simulink model "Aerial_Inspection_Octa_Rotor"  (R2021a)
settings: Solver=VariableStepAuto  StartTime=0.0  StopTime=2  RelTol=1e-3
model workspace: external: MATLAB File D:\MS_Control_Project\Simulation\SolidWorks output\Aerial_Inspection_Octa_Rotor_DataFile.m (data not in the file)
undefined symbols (not defined in the file or in its folder): Motor_data, params, servo_specs, smiData, stepper, Tm, X, Y, Z
libraries: sm_lib x810, nesl_utility x50, sharedtransform x1
(part 4 of 21)

== system Aerial_Inspection_Octa_Rotor/UAV/Device ==
  Device_1_RIGID : Subsystem
  Device_Box_1_RIGID : Subsystem
  F : PMIOPort  Side=Left
  connections:
  Device_1_RIGID/LConn1 -- Device_Box_1_RIGID/LConn1
  Device_Box_1_RIGID/LConn2 -- F/RConn1

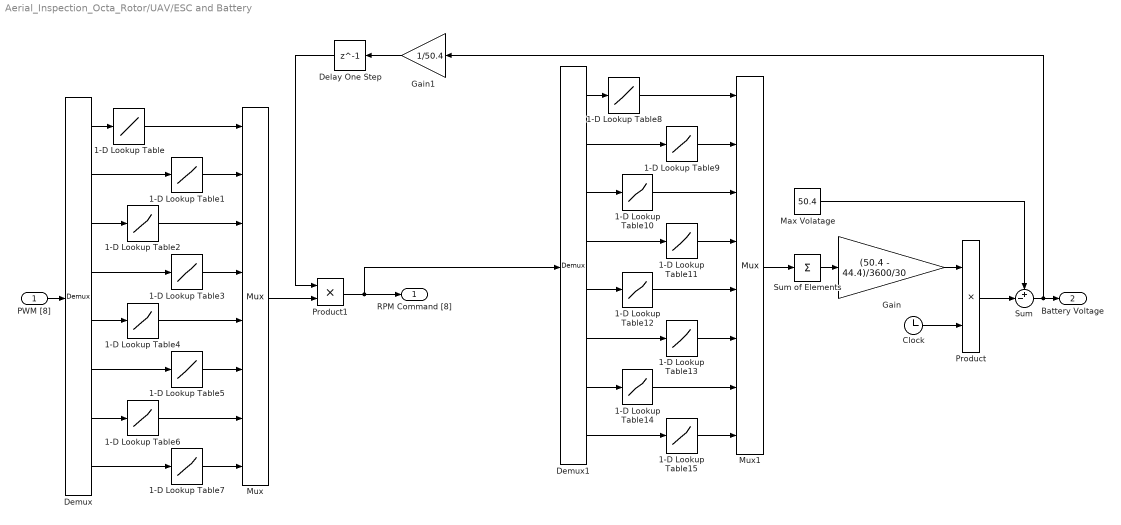
== system Aerial_Inspection_Octa_Rotor/UAV/ESC and Battery ==
  PWM [8] : Inport
  1-D Lookup Table{,1..7} (8 alike) : Lookup_n-D  NumberOfTableDimensions=1  BreakpointsForDimension1=[0;Motor_data.Throttle]  Table=[0;Motor_data.RPM]  InternalRulePriority=Speed  RndMeth=Simplest  InputSameDT=on
  1-D Lookup Table{8..15} (8 alike) : Lookup_n-D  NumberOfTableDimensions=1  BreakpointsForDimension1=[0;Motor_data.RPM]  Table=[0;Motor_data.Current]  InterpMethod=Cubic spline  ExtrapMethod=Cubic spline  InternalRulePriority=Speed  RndMeth=Simplest  InputSameDT=on
  Clock : Clock
  Delay One Step : Delay  DelayLength=1  InitialCondition=50.4
  Demux : Demux  Outputs=8
  Demux1 : Demux  Outputs=8
  Gain : Gain  Gain=(50.4 - 44.4)/3600/30
  Gain1 : Gain  Gain=1/50.4
  Max Volatage : Constant  Value=50.4
  Mux : Mux  Inputs=8
  Mux1 : Mux  Inputs=8
  Product : Product
  Product1 : Product
  Sum : Sum  Inputs=+-|
  Sum of Elements : Sum  Inputs=+
  RPM Command [8] : Outport
  Battery Voltage : Outport  Port=2
  wires:
  PWM [8]/1 -> Demux/1
  Demux/1 -> 1-D Lookup Table/1
  Demux/2 -> 1-D Lookup Table1/1
  Demux/3 -> 1-D Lookup Table2/1
  Demux/4 -> 1-D Lookup Table3/1
  Demux/5 -> 1-D Lookup Table4/1
  Demux/6 -> 1-D Lookup Table5/1
  Demux/7 -> 1-D Lookup Table6/1
  Demux/8 -> 1-D Lookup Table7/1
  1-D Lookup Table7/1 -> Mux/8
  1-D Lookup Table5/1 -> Mux/6
  1-D Lookup Table3/1 -> Mux/4
  1-D Lookup Table1/1 -> Mux/2
  1-D Lookup Table6/1 -> Mux/7
  1-D Lookup Table4/1 -> Mux/5
  1-D Lookup Table2/1 -> Mux/3
  1-D Lookup Table/1 -> Mux/1
  1-D Lookup Table8/1 -> Mux1/1
  1-D Lookup Table10/1 -> Mux1/3
  1-D Lookup Table12/1 -> Mux1/5
  1-D Lookup Table14/1 -> Mux1/7
  1-D Lookup Table9/1 -> Mux1/2
  1-D Lookup Table11/1 -> Mux1/4
  1-D Lookup Table13/1 -> Mux1/6
  1-D Lookup Table15/1 -> Mux1/8
  Demux1/8 -> 1-D Lookup Table15/1
  Demux1/7 -> 1-D Lookup Table14/1
  Demux1/6 -> 1-D Lookup Table13/1
  Demux1/5 -> 1-D Lookup Table12/1
  Demux1/4 -> 1-D Lookup Table11/1
  Demux1/3 -> 1-D Lookup Table10/1
  Demux1/2 -> 1-D Lookup Table9/1
  Demux1/1 -> 1-D Lookup Table8/1
  Mux1/1 -> Sum of Elements/1
  Sum of Elements/1 -> Gain/1
  Product/1 -> Sum/2
  Gain/1 -> Product/1
  Clock/1 -> Product/2
  Max Volatage/1 -> Sum/1
  Sum/1 -> Gain1/1, Battery Voltage/1
  Mux/1 -> Product1/2
  Product1/1 -> Demux1/1, RPM Command [8]/1
  Gain1/1 -> Delay One Step/1
  Delay One Step/1 -> Product1/1

== system Aerial_Inspection_Octa_Rotor/UAV/Landing Gear ==
  Front_lastic_1_RIGID : Subsystem
  Front_lastic_2_RIGID : Subsystem
  Landing_Gear_5_RIGID : Subsystem
  Rear_lastic_1_RIGID : Subsystem
  Rear_lastic_2_RIGID : Subsystem
  Revolute16 : sm_lib/Joints/Revolute Joint  JointMode=Normal  SenseConstraintForce=off  SenseConstraintForceX=off  SenseConstraintForceY=off  SenseConstraintForceZ=off  SenseConstraintTorque=off  SenseConstraintTorqueX=off  SenseConstraintTorqueY=off  SenseConstraintTorqueZ=off  SenseTotalForce=off  SenseTotalForceX=off  SenseTotalForceY=off  SenseTotalForceZ=off  SenseTotalTorque=off  SenseTotalTorqueX=off  SenseTotalTorqueY=off  SenseTotalTorqueZ=off  CompositeWrenchDir=FollowerOnBase  CompositeWrenchFrame=BaseFrame  EquilibriumPosition=0  EquilibriumPositionUnits=deg  SpringStiffness=0  SpringStiffnessUnits=N*m/deg  DampingCoefficient=0  DampingCoefficientUnits=N*m/(deg/s)  TorqueActuationMode=NoTorque  MotionActuationMode=ComputedMotion  SensePosition=off  SenseVelocity=off  SenseAcceleration=off  SenseTorqueForce=off  SenseLowerLimitTorqueForce=off  SenseUpperLimitTorqueForce=off  LowerLimitSpecify=off  LowerLimitBound=-90  LowerLimitBoundUnits=deg  LowerLimitStiffness=1e4  LowerLimitStiffnessUnits=N*m/deg  LowerLimitDamping=10  LowerLimitDampingUnits=N*m/(deg/s)  LowerLimitTransitionRegionWidth=0.1  LowerLimitTransitionRegionWidthUnits=deg  UpperLimitSpecify=off  UpperLimitBound=90  UpperLimitBoundUnits=deg  UpperLimitStiffness=1e4  UpperLimitStiffnessUnits=N*m/deg  UpperLimitDamping=10  UpperLimitDampingUnits=N*m/(deg/s)  UpperLimitTransitionRegionWidth=0.1  UpperLimitTransitionRegionWidthUnits=deg  PositionTargetSpecify=on  PositionTargetPriority=Low  PositionTargetValue=smiData.RevoluteJoint(17).Rz.Pos  PositionTargetValueUnits=deg  VelocityTargetSpecify=off  VelocityTargetPriority=High  VelocityTargetValue=0  VelocityTargetValueUnits=deg/s
  Revolute17 : sm_lib/Joints/Revolute Joint  JointMode=Normal  SenseConstraintForce=off  SenseConstraintForceX=off  SenseConstraintForceY=off  SenseConstraintForceZ=off  SenseConstraintTorque=off  SenseConstraintTorqueX=off  SenseConstraintTorqueY=off  SenseConstraintTorqueZ=off  SenseTotalForce=off  SenseTotalForceX=off  SenseTotalForceY=off  SenseTotalForceZ=off  SenseTotalTorque=off  SenseTotalTorqueX=off  SenseTotalTorqueY=off  SenseTotalTorqueZ=off  CompositeWrenchDir=FollowerOnBase  CompositeWrenchFrame=BaseFrame  EquilibriumPosition=0  EquilibriumPositionUnits=deg  SpringStiffness=0  SpringStiffnessUnits=N*m/deg  DampingCoefficient=0  DampingCoefficientUnits=N*m/(deg/s)  TorqueActuationMode=NoTorque  MotionActuationMode=ComputedMotion  SensePosition=off  SenseVelocity=off  SenseAcceleration=off  SenseTorqueForce=off  SenseLowerLimitTorqueForce=off  SenseUpperLimitTorqueForce=off  LowerLimitSpecify=off  LowerLimitBound=-90  LowerLimitBoundUnits=deg  LowerLimitStiffness=1e4  LowerLimitStiffnessUnits=N*m/deg  LowerLimitDamping=10  LowerLimitDampingUnits=N*m/(deg/s)  LowerLimitTransitionRegionWidth=0.1  LowerLimitTransitionRegionWidthUnits=deg  UpperLimitSpecify=off  UpperLimitBound=90  UpperLimitBoundUnits=deg  UpperLimitStiffness=1e4  UpperLimitStiffnessUnits=N*m/deg  UpperLimitDamping=10  UpperLimitDampingUnits=N*m/(deg/s)  UpperLimitTransitionRegionWidth=0.1  UpperLimitTransitionRegionWidthUnits=deg  PositionTargetSpecify=on  PositionTargetPriority=Low  PositionTargetValue=smiData.RevoluteJoint(18).Rz.Pos  PositionTargetValueUnits=deg  VelocityTargetSpecify=off  VelocityTargetPriority=High  VelocityTargetValue=0  VelocityTargetValueUnits=deg/s
  Revolute4 : sm_lib/Joints/Revolute Joint  JointMode=Normal  SenseConstraintForce=off  SenseConstraintForceX=off  SenseConstraintForceY=off  SenseConstraintForceZ=off  SenseConstraintTorque=off  SenseConstraintTorqueX=off  SenseConstraintTorqueY=off  SenseConstraintTorqueZ=off  SenseTotalForce=off  SenseTotalForceX=off  SenseTotalForceY=off  SenseTotalForceZ=off  SenseTotalTorque=off  SenseTotalTorqueX=off  SenseTotalTorqueY=off  SenseTotalTorqueZ=off  CompositeWrenchDir=FollowerOnBase  CompositeWrenchFrame=BaseFrame  EquilibriumPosition=0  EquilibriumPositionUnits=deg  SpringStiffness=0  SpringStiffnessUnits=N*m/deg  DampingCoefficient=0  DampingCoefficientUnits=N*m/(deg/s)  TorqueActuationMode=NoTorque  MotionActuationMode=ComputedMotion  SensePosition=off  SenseVelocity=off  SenseAcceleration=off  SenseTorqueForce=off  SenseLowerLimitTorqueForce=off  SenseUpperLimitTorqueForce=off  LowerLimitSpecify=off  LowerLimitBound=-90  LowerLimitBoundUnits=deg  LowerLimitStiffness=1e4  LowerLimitStiffnessUnits=N*m/deg  LowerLimitDamping=10  LowerLimitDampingUnits=N*m/(deg/s)  LowerLimitTransitionRegionWidth=0.1  LowerLimitTransitionRegionWidthUnits=deg  UpperLimitSpecify=off  UpperLimitBound=90  UpperLimitBoundUnits=deg  UpperLimitStiffness=1e4  UpperLimitStiffnessUnits=N*m/deg  UpperLimitDamping=10  UpperLimitDampingUnits=N*m/(deg/s)  UpperLimitTransitionRegionWidth=0.1  UpperLimitTransitionRegionWidthUnits=deg  PositionTargetSpecify=on  PositionTargetPriority=Low  PositionTargetValue=smiData.RevoluteJoint(5).Rz.Pos  PositionTargetValueUnits=deg  VelocityTargetSpecify=off  VelocityTargetPriority=High  VelocityTargetValue=0  VelocityTargetValueUnits=deg/s
  Revolute5 : sm_lib/Joints/Revolute Joint  JointMode=Normal  SenseConstraintForce=off  SenseConstraintForceX=off  SenseConstraintForceY=off  SenseConstraintForceZ=off  SenseConstraintTorque=off  SenseConstraintTorqueX=off  SenseConstraintTorqueY=off  SenseConstraintTorqueZ=off  SenseTotalForce=off  SenseTotalForceX=off  SenseTotalForceY=off  SenseTotalForceZ=off  SenseTotalTorque=off  SenseTotalTorqueX=off  SenseTotalTorqueY=off  SenseTotalTorqueZ=off  CompositeWrenchDir=FollowerOnBase  CompositeWrenchFrame=BaseFrame  EquilibriumPosition=0  EquilibriumPositionUnits=deg  SpringStiffness=0  SpringStiffnessUnits=N*m/deg  DampingCoefficient=0  DampingCoefficientUnits=N*m/(deg/s)  TorqueActuationMode=NoTorque  MotionActuationMode=ComputedMotion  SensePosition=off  SenseVelocity=off  SenseAcceleration=off  SenseTorqueForce=off  SenseLowerLimitTorqueForce=off  SenseUpperLimitTorqueForce=off  LowerLimitSpecify=off  LowerLimitBound=-90  LowerLimitBoundUnits=deg  LowerLimitStiffness=1e4  LowerLimitStiffnessUnits=N*m/deg  LowerLimitDamping=10  LowerLimitDampingUnits=N*m/(deg/s)  LowerLimitTransitionRegionWidth=0.1  LowerLimitTransitionRegionWidthUnits=deg  UpperLimitSpecify=off  UpperLimitBound=90  UpperLimitBoundUnits=deg  UpperLimitStiffness=1e4  UpperLimitStiffnessUnits=N*m/deg  UpperLimitDamping=10  UpperLimitDampingUnits=N*m/(deg/s)  UpperLimitTransitionRegionWidth=0.1  UpperLimitTransitionRegionWidthUnits=deg  PositionTargetSpecify=on  PositionTargetPriority=Low  PositionTargetValue=smiData.RevoluteJoint(6).Rz.Pos  PositionTargetValueUnits=deg  VelocityTargetSpecify=off  VelocityTargetPriority=High  VelocityTargetValue=0  VelocityTargetValueUnits=deg/s
  F : PMIOPort  Side=Left
  connections:
  Front_lastic_2_RIGID/LConn1 -- Revolute17/RConn1
  Landing_Gear_5_RIGID/RConn3 -- Revolute5/LConn1
  Landing_Gear_5_RIGID/RConn1 -- Revolute17/LConn1
  Landing_Gear_5_RIGID/RConn2 -- Revolute16/LConn1
  Rear_lastic_1_RIGID/LConn1 -- Revolute4/RConn1
  Front_lastic_1_RIGID/LConn1 -- Revolute16/RConn1
  Rear_lastic_2_RIGID/LConn1 -- Revolute5/RConn1
  Landing_Gear_5_RIGID/RConn4 -- Revolute4/LConn1
  F/RConn1 -- Landing_Gear_5_RIGID/LConn1
